simulink model "FSKMethod1"  (R2019b)
settings: Solver=VariableStepAuto  StartTime=0.0  StopTime=10  RelTol=1e-3
libraries: commsynccomp2 x1
settings Model: Creator=z3454314  LastModifiedBy=z3454314

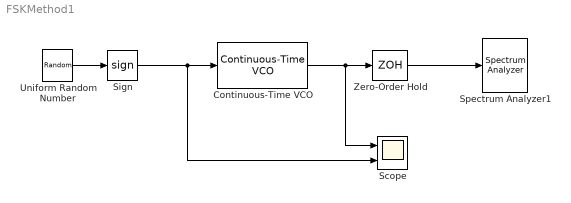
== system FSKMethod1 ==
  Continuous-Time VCO : commsynccomp2/Continuous-Time VCO  Ac=1  Fc=8000  Kc=2000  Ph=0
      settings: SourceProductName=Communications Toolbox  SourceProductBaseCode=CM
  Scope : Scope  NumInputPorts=2
  Sign : Signum
  Spectrum Analyzer1 : SpectrumAnalyzer
  Uniform Random Number : UniformRandomNumber  SampleTime=1/2000
  Zero-Order Hold : ZeroOrderHold  SampleTime=1/44100
  wires:
  Uniform Random Number/1 -> Sign/1
  Sign/1 -> Scope/2, Continuous-Time VCO/1
  Zero-Order Hold/1 -> Spectrum Analyzer1/1
  Continuous-Time VCO/1 -> Scope/1, Zero-Order Hold/1
